simulink model "speedcontrol"  (R2022b)
settings: Solver=VariableStepAuto  StartTime=0.0  StopTime=1  MaxStep=1e-6  RelTol=1e-6
InitFcn:
  | Ra=0.5;
  | La=2.5e-3;
  | Kc=0.35;
  | Ke=0.35;
  | J=1e-3;
  | alphac=2*pi*500;
  | kpc=alphac*La;
  | Kic=alphac*2*La;
  | r=kpc-Ra;
  | Umax=140;
  | Umin=-140;
libraries: simulink x1, slpidlib x1
settings Model: Creator=User  LastModifiedBy=richa
settings ModelReferenceCC: EnableRefExpFcnMdlSchedulingChecks=on

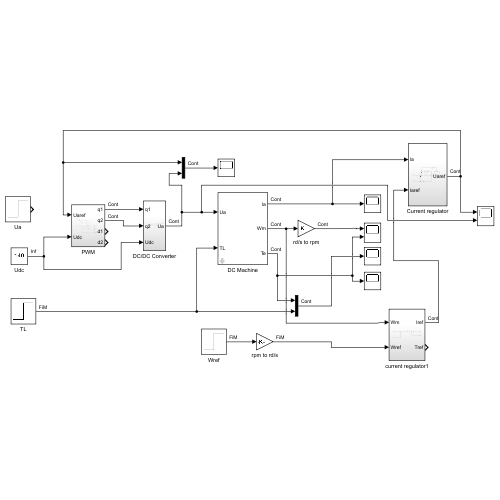
[thumbnail: Simulink's stored preview of the top-level diagram]
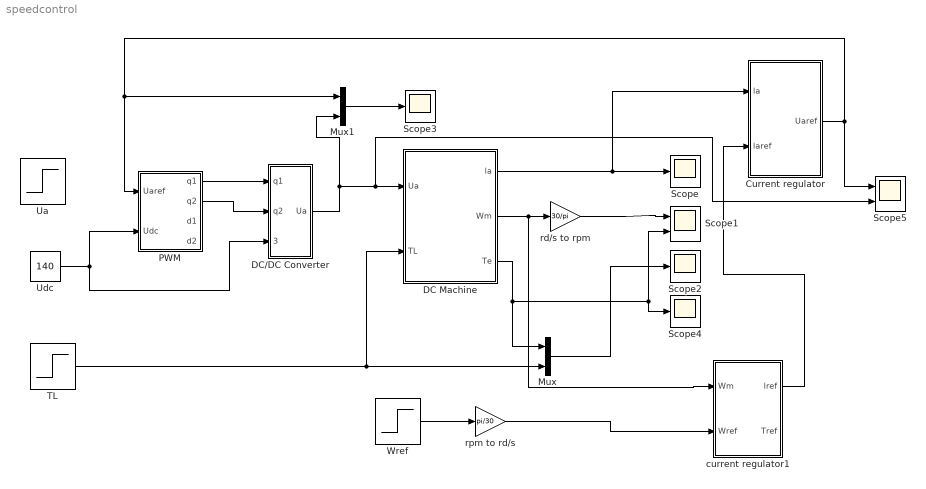
== system speedcontrol ==
  Current regulator : Subsystem
  DC Machine : Subsystem  mask{Ra=0.5, La=2.5e-3, J=1e-3, fr=5e-2, Ke=0.35, Kc=0.35}
      mask prompts: Ra "Ra(Ohm)"; La "La(H)"; J "J(N.m.s^-1)"; fr "fr(N.m.s)"; Ke "Ke(V.s)"; Kc "Kc(N.m.A^-1)"
  DC/DC Converter : Subsystem
  Mux : Mux  Inputs=2
  Mux1 : Mux  Inputs=2
  PWM : Subsystem
  Scope{,2..4} (4 alike) : Scope
  Scope1 : Scope  NumInputPorts=2
  Scope5 : Scope  NumInputPorts=2
  TL : Step  Time=0.5  After=7  SampleTime=0
  Ua : Step  Time=0.1  After=120  SampleTime=0
  Udc : Constant  Value=140
  Wref : Step  Time=0.1  After=2000  SampleTime=0
  current regulator1 : Subsystem
  rd/s to rpm : Gain  Gain=30/pi
  rpm to rd/s : Gain  Gain=pi/30
  wires:
  DC Machine/2(Wm) -> current regulator1/1(Wm), rd/s to rpm/1
  PWM/1(q1) -> DC/DC Converter/1(q1)
  PWM/2(q2) -> DC/DC Converter/2(q2)
  DC/DC Converter/1(Ua) -> Mux1/2, Scope5/2, DC Machine/1(Ua)
  TL/1 -> Mux/2, DC Machine/2(TL)
  Udc/1 -> DC/DC Converter/3(Udc), PWM/2(Udc)
  Mux/1 -> Scope2/1
  Mux1/1 -> Scope3/1
  rd/s to rpm/1 -> Scope1/1
  Wref/1 -> rpm to rd/s/1
  rpm to rd/s/1 -> current regulator1/2(Wref)
  current regulator1/1(lref) -> Current regulator/2(laref)
  DC Machine/1(la) -> Current regulator/1(la), Scope/1
  Current regulator/1(Uaref) -> Mux1/1, PWM/1(Uaref), Scope5/1
  DC Machine/3(Te) -> Mux/1, Scope1/2, Scope4/1

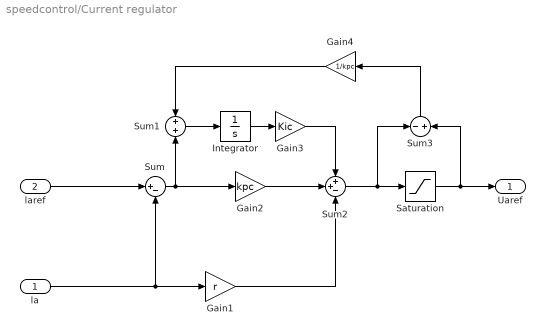
== system speedcontrol/Current regulator ==
  la : Inport
  laref : Inport  Port=2
  Gain1 : Gain  Gain=r
  Gain2 : Gain  Gain=kpc
  Gain3 : Gain  Gain=Kic
  Gain4 : Gain  Gain=1/kpc
  Integrator : Integrator
  Saturation : Saturate  UpperLimit=Umax  LowerLimit=-Umax
  Sum : Sum  Inputs=|+-
  Sum1 : Sum  Inputs=+|+
  Sum2 : Sum  Inputs=++-
  Sum3 : Sum  Inputs=-|+
  Uaref : Outport
  wires:
  la/1 -> Gain1/1, Sum/2
  laref/1 -> Sum/1
  Sum/1 -> Sum1/2, Gain2/1
  Sum1/1 -> Integrator/1
  Integrator/1 -> Gain3/1
  Gain2/1 -> Sum2/2
  Gain3/1 -> Sum2/1
  Gain1/1 -> Sum2/3
  Saturation/1 -> Sum3/2, Uaref/1
  Sum2/1 -> Sum3/1, Saturation/1
  Gain4/1 -> Sum1/1
  Sum3/1 -> Gain4/1

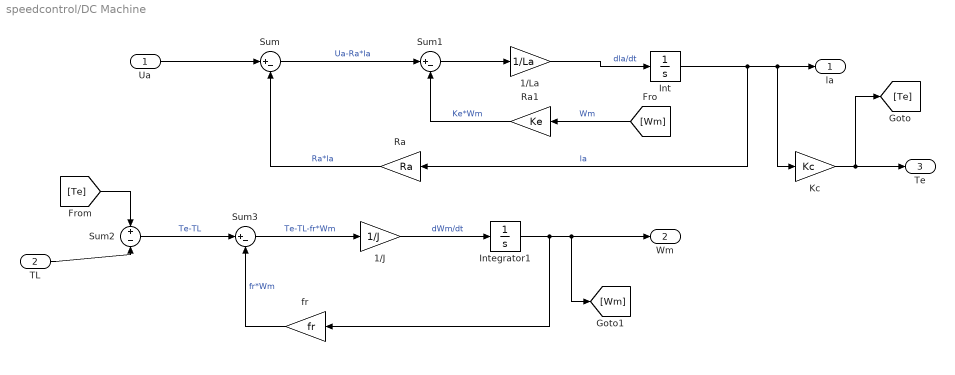
== system speedcontrol/DC Machine ==
  Ua : Inport
  TL : Inport  Port=2
  1/J : Gain  Gain=1/J
  1/La : Gain  Gain=1/La
  Int : Integrator
  Integrator1 : Integrator
  Kc : Gain  Gain=Kc
  Ra : Gain  Gain=Ra
  Ra1 : Gain  Gain=Ke
  Sum : Sum  Inputs=|+-
  Sum1 : Sum  Inputs=|+-
  Sum2 : Sum  Inputs=+-
  Sum3 : Sum  Inputs=|+-
  fr : Gain  Gain=fr
  la : Outport
  Wm : Outport  Port=2
  Te : Outport  Port=3
  wires:
  [Wm] -> Ra1/1  "Wm"
  Sum1/1 -> 1/La/1
  Ra1/1 -> Sum1/2  "Ke*Wm"
  Kc/1 -> Te/1, [Te]
  1/J/1 -> Integrator1/1  "dWm/dt"
  Ra/1 -> Sum/2  "Ra*la"
  Integrator1/1 -> fr/1, Wm/1, [Wm]
  fr/1 -> Sum3/2  "fr*Wm"
  Sum3/1 -> 1/J/1  "Te-TL-fr*Wm"
  Sum2/1 -> Sum3/1  "Te-TL"
  Int/1 -> Ra/1, la/1, Kc/1  "la"
  TL/1 -> Sum2/2
  1/La/1 -> Int/1  "dla/dt"
  Ua/1 -> Sum/1
  Sum/1 -> Sum1/1  "Ua-Ra*la"
  [Te] -> Sum2/1

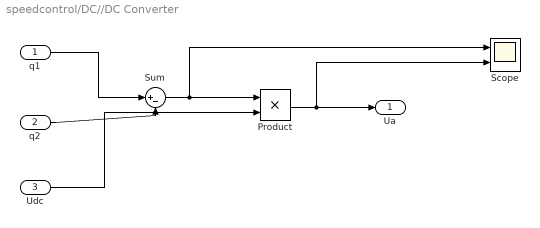
== system speedcontrol/DC//DC Converter ==
  q1 : Inport
  q2 : Inport  Port=2
  Udc : Inport  Port=3
  Product : Product
  Scope : Scope  NumInputPorts=2
  Sum : Sum  Inputs=|+-
  Ua : Outport
  wires:
  q1/1 -> Sum/1
  q2/1 -> Sum/2
  Udc/1 -> Product/2
  Sum/1 -> Scope/1, Product/1
  Product/1 -> Scope/2, Ua/1

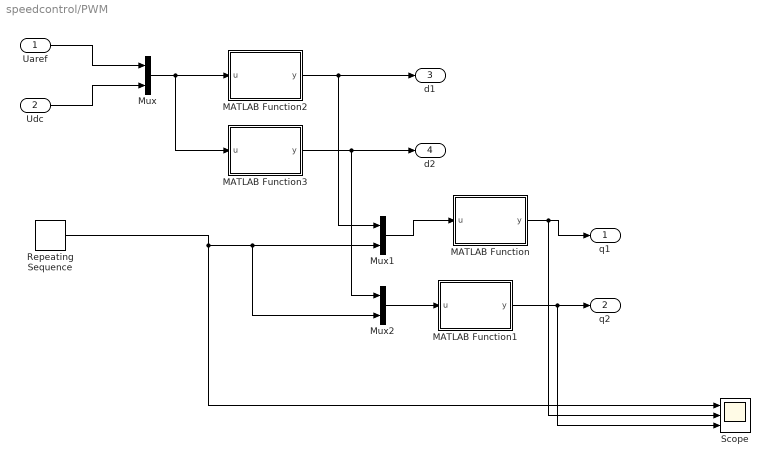
== system speedcontrol/PWM ==
  Uaref : Inport
  Udc : Inport  Port=2
  MATLAB Function : MATLAB Function  TreatAsAtomicUnit=on
  MATLAB Function1 : MATLAB Function  TreatAsAtomicUnit=on
  MATLAB Function2 : MATLAB Function  TreatAsAtomicUnit=on
  MATLAB Function3 : MATLAB Function  TreatAsAtomicUnit=on
  Mux : Mux  Inputs=2
  Mux1 : Mux  Inputs=2
  Mux2 : Mux  Inputs=2
  Repeating Sequence : simulink/Sources/Repeating Sequence  rep_seq_t=[0 100e-6 200e-6]  rep_seq_y=[1 0 1]
  Scope : Scope  NumInputPorts=3
  q1 : Outport
  q2 : Outport  Port=2
  d1 : Outport  Port=3
  d2 : Outport  Port=4
  wires:
  Uaref/1 -> Mux/1
  Udc/1 -> Mux/2
  Mux/1 -> MATLAB Function3/1(u), MATLAB Function2/1(u)
  MATLAB Function3/1(y) -> Mux2/1, d2/1
  MATLAB Function2/1(y) -> Mux1/1, d1/1
  Mux2/1 -> MATLAB Function1/1(u)
  Mux1/1 -> MATLAB Function/1(u)
  MATLAB Function/1(y) -> Scope/2, q1/1
  MATLAB Function1/1(y) -> Scope/3, q2/1
  Repeating Sequence/1 -> Scope/1, Mux2/2, Mux1/2

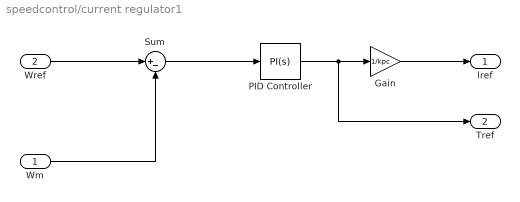
== system speedcontrol/current regulator1 ==
  Wm : Inport
  Wref : Inport  Port=2
  Gain : Gain  Gain=1/kpc
  PID Controller : slpidlib/PID Controller  Controller=PI  Form=Parallel  TimeDomain=Continuous-time  UseExternalTs=off  SampleTime=-1  IntegratorMethod=Forward Euler  FilterMethod=Forward Euler  ControllerParametersSource=internal  P=5  I=0.1  UseKiTs=off  D=0  N=100  UseFilter=on  TunerSelectOption=Transfer Function Based (PID Tuner App)  InitialConditionSource=internal  InitialConditionForIntegrator=0  InitialConditionForFilter=0  DifferentiatorICPrevScaledInput=0  ExternalReset=none  TrackingMode=off  Kt=1  LimitOutput=off  SatLimitsSource=internal  UpperSaturationLimit=inf  LowerSaturationLimit=-inf  LinearizeAsGain=on  AntiWindupMode=none  Kb=1  LimitIntegrator=off  UpperIntegratorSaturationLimit=inf  LowerIntegratorSaturationLimit=-inf  POutMin=[]  POutMax=[]  IOutMin=[]  IOutMax=[]  DOutMin=[]  DOutMax=[]  NOutMin=[]  NOutMax=[]  SumOutMin=[]  SumOutMax=[]  SaturationOutMin=[]  SaturationOutMax=[]  PParamMin=[]  PParamMax=[]  IParamMin=[]  IParamMax=[]  DParamMin=[]  DParamMax=[]  NParamMin=[]  NParamMax=[]  KbParamMin=[]  KbParamMax=[]  KtParamMin=[]  KtParamMax=[]  KbOutMin=[]  KbOutMax=[]  KtOutMin=[]  KtOutMax=[]  IntegratorOutMin=[]  IntegratorOutMax=[]  FilterOutMin=[]  FilterOutMax=[]  SumI1OutMin=[]  SumI1OutMax=[]  SumI2OutMin=[]  SumI2OutMax=[]  SumI3OutMin=[]  SumI3OutMax=[]  SumI4OutMin=[]  SumI4OutMax=[]  SumDOutMin=[]  SumDOutMax=[]  DifferentiatorOutMin=[]  DifferentiatorOutMax=[]  FilterDiffOutCoefMin=[]  FilterDiffOutCoefMax=[]  ReciprocalOutMin=[]  ReciprocalOutMax=[]  SumDenOutMin=[]  SumDenOutMax=[]  SumNumOutMin=[]  SumNumOutMax=[]  DivideOutMin=[]  DivideOutMax=[]  UdiffTsProdOutMin=[]  UdiffTsProdOutMax=[]  NTsProdOutMin=[]  NTsProdOutMax=[]  UintegralTsProdOutMin=[]  UintegralTsProdOutMax=[]  UngainTsProdOutMin=[]  UngainTsProdOutMax=[]  ClampingZeroOutDataTypeStr=Inherit: Inherit via back propagation  ClampingZeroOutMin=[]  ClampingZeroOutMax=[]  FilterDenConstantOutDataTypeStr=Inherit: Inherit via back propagation  FilterDenConstantOutMin=[]  FilterDenConstantOutMax=[]  PCopyOutDataTypeStr=Inherit: Inherit via back propagation  PCopyOutMin=[]  PCopyOutMax=[]  NCopyOutDataTypeStr=Inherit: Inherit via back propagation  NCopyOutMin=[]  NCopyOutMax=[]  IntegratorContinuousStateAttributes=''  IntegratorStateMustResolveToSignalObject=off  IntegratorRTWStateStorageClass=Auto  FilterContinuousStateAttributes=''  FilterStateMustResolveToSignalObject=off  FilterRTWStateStorageClass=Auto  ParallelPVariant=InternalParameters  IdealPVariant=Disabled  IVariant=InternalParameters  DVariant=Disabled  IntegratorVariant=Continuous  SatVariant=Disabled  AWVariant=Passthrough  PCopyVariant=Disabled  TRVariant=Disabled  FdbkBlocksVariant=Forward  IdealPFdbkVariant=Disabled  SatFdbkVariant=Disabled  DerivativeFilterVariant=Disabled  NVariant=Disabled  NCopyVariant=Disabled_SignalSpec  FilterICVariant=Disabled  IntegratorICVariant=InternalICs  ExternalResetVariant=Disabled  TRSumVariant=Passthrough  SumFdbkVariant=Disabled  SumVariant=Sum_PI  TsampFilterVariant=InternalTs  TsampNgainVariant=Passthrough  TsampIntegralVariant=Passthrough  ExternalSaturationOutDataTypeStr=Inherit: Same as second input
  Sum : Sum  Inputs=|+-
  lref : Outport
  Tref : Outport  Port=2
  wires:
  Wref/1 -> Sum/1
  Wm/1 -> Sum/2
  Sum/1 -> PID Controller/1
  PID Controller/1 -> Tref/1, Gain/1
  Gain/1 -> lref/1

== matlab function speedcontrol/PWM/MATLAB Function ==
  data: u input; y output
function y=fcn(u)

y=(u(1)>u(2));

== matlab function speedcontrol/PWM/MATLAB Function2 ==
  data: u input; y output
function y=fcn(u)

y=(0.5*(1+u(1)/u(2)));

== matlab function speedcontrol/PWM/MATLAB Function3 ==
  data: u input; y output
function y=fcn(u)

y=(0.5*(1-u(1)/u(2)));

== matlab function speedcontrol/PWM/MATLAB Function1 ==
  data: u input; y output
function y=fcn(u)

y=(u(1)>u(2));
